simulink model "P3_test_sim"  (R2019a)
settings: Solver=VariableStepAuto  StartTime=0.0  StopTime=10.0  RelTol=1e-3
values from neighbouring files (symbols this model uses):
  A_AA = [ybb  yp+w0/u0 yr-1 g*ctt0/u0 ... (first row only)    [P1.m]    (also in P2.m; P3.m; P3_F.m; P3_serv.m)
  B = [0    ydr ... (first row only)    [P1.m]    (also in P2.m; P3.m; P3_F.m; P3_serv.m)
  bb_ref = 3    [P3.m]    (also in P3_F.m = 0.8; P3_serv.m = 0.8; P3_test.m; P4_F.m = 0.8)
  bb_stept = 10    [P3.m]    (also in P3_F.m; P3_serv.m; P3_test.m; P4_F.m)
  C = eye(4)    [P2.m]    (also in P3.m; P3_F.m; P3_serv.m; P3_test.m)
  D = zeros(4,2)    [P2.m]    (also in P3.m; P3_F.m; P3_serv.m; P3_test.m)
  deg = pi/180    (= 0.0174532925199)    [P1.m]    (also in P2.m; P3.m; P3_F.m; P3_serv.m)
  F = (CC*dcgain)^(-1)    [P3_F.m]    (also in P3_test.m; P4_F.m; P5.m; P5_F.m)
  K_lqr = lqr(A2_AA,B2,Q,R)    [P3.m]    (also in P3_F.m = lqr(A_AA,B,Q,R); P3_serv.m; P3_test.m = lqr(A_AA,B,Q,R); P4_F.m = lqr(A_AA,B,Q,R))
  phi_ref = 8    [P3.m]    (also in P3_F.m = 15; P3_serv.m; P3_test.m; P4_F.m = 22)
  phi_stept = 50    [P3.m]    (also in P3_F.m; P3_serv.m; P3_test.m; P4_F.m)
settings Model: Creator=tomas  LastModifiedBy=tomas

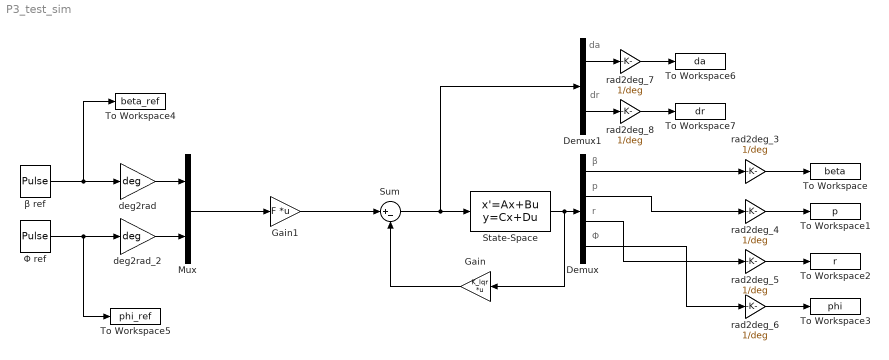
== system P3_test_sim ==
  note: da
  note: dr
  note: p
  note: r
  note: Φ
  note: β
  Demux : Demux
  Demux1 : Demux  Outputs=2
  Gain : Gain  Gain=K_lqr  Multiplication=Matrix(K*u) (u vector)
  Gain1 : Gain  Gain=F  Multiplication=Matrix(K*u) (u vector)
  Mux : Mux  Inputs=2
  State-Space : StateSpace  A=A_AA  B=B  C=C  D=D  InitialCondition=0
  Sum : Sum  Inputs=|+-
  To Workspace : ToWorkspace  VariableName=beta  SaveFormat=Timeseries  SampleTime=-1
  To Workspace1 : ToWorkspace  VariableName=p  SaveFormat=Timeseries  SampleTime=-1
  To Workspace2 : ToWorkspace  VariableName=r  SaveFormat=Timeseries  SampleTime=-1
  To Workspace3 : ToWorkspace  VariableName=phi  SaveFormat=Timeseries  SampleTime=-1
  To Workspace4 : ToWorkspace  VariableName=beta_ref  SaveFormat=Timeseries  SampleTime=-1
  To Workspace5 : ToWorkspace  VariableName=phi_ref  SaveFormat=Timeseries  SampleTime=-1
  To Workspace6 : ToWorkspace  VariableName=da  SaveFormat=Timeseries  SampleTime=-1
  To Workspace7 : ToWorkspace  VariableName=dr  SaveFormat=Timeseries  SampleTime=-1
  deg2rad : Gain  Gain=deg
  deg2rad_2 : Gain  Gain=deg
  rad2deg_{3..8} (6 alike) : Gain  Gain=1/deg
  Φ ref : DiscretePulseGenerator  PulseType=Time based  Amplitude=phi_ref  Period=100  PulseWidth=20  PhaseDelay=phi_stept
  β ref : DiscretePulseGenerator  PulseType=Time based  Amplitude=bb_ref  Period=100  PulseWidth=20  PhaseDelay=bb_stept
  wires:
  Demux1/2 -> rad2deg_8/1
  rad2deg_6/1 -> To Workspace3/1
  rad2deg_5/1 -> To Workspace2/1
  rad2deg_3/1 -> To Workspace/1
  rad2deg_4/1 -> To Workspace1/1
  Demux1/1 -> rad2deg_7/1
  Φ ref/1 -> deg2rad_2/1, To Workspace5/1
  Demux/3 -> rad2deg_5/1
  rad2deg_7/1 -> To Workspace6/1
  deg2rad/1 -> Mux/1
  deg2rad_2/1 -> Mux/2
  rad2deg_8/1 -> To Workspace7/1
  Sum/1 -> State-Space/1, Demux1/1
  Demux/4 -> rad2deg_6/1
  State-Space/1 -> Gain/1, Demux/1
  Demux/1 -> rad2deg_3/1
  β ref/1 -> To Workspace4/1, deg2rad/1
  Demux/2 -> rad2deg_4/1
  Gain/1 -> Sum/2
  Mux/1 -> Gain1/1
  Gain1/1 -> Sum/1
